simulink model "substation"  (R2023b)
settings: Solver=VariableStepAuto  StartTime=0.0  StopTime=1  FixedStep=1/48000  MaxStep=1e-3  RelTol=1e-3  EnableMultiTasking=on
libraries: spsGroundLib x4, spsThreePhaseBreakerLib x3, spsSurgeArresterLib x3, spsThreePhaseVIMeasurementLib x2, spsThreePhaseParallelRLCLoadLib x1, spsThreePhaseDynamicLoadLib x1, spsThreePhaseProgrammableVoltageSourceLib x1, dspnetwork x1, spsThreePhaseTransformerTwoWindingsLib x1, sps_lib x1
settings Model: SimulationMode=rapid-accelerator  Creator=foo  LastModifiedBy=shaow
settings SolverCC: AlgebraicLoopSolver=TrustRegion  AutoInsertRateTranBlk=on  MaxZcPerStep=1
settings DataIOCC: LimitDataPoints=on  MaxDataPoints=10000  SaveOutput=off  DSMLogging=off  SaveTime=off
settings OptimizationCC: ReuseModelBlockBuffer=off  LifeSpan=inf  SimCompilerOptimization=on
settings DebuggingCC: UnconnectedInputMsg=warning  UnconnectedOutputMsg=warning  UnconnectedLineMsg=warning  AllowSymbolicDim=off  SFUnexpectedBacktrackingDiag=warning  SFNoUnconditionalDefaultTransitionDiag=warning  SFExecutionAtInitializationDiag=none  ArithmeticOperatorsInVariantConditions=warning
settings ModelReferenceCC: EnableRefExpFcnMdlSchedulingChecks=on
settings SFSimCC: SimUseLocalCustomCode=off  CustomCodeUndefinedFunction=UseInterfaceOnly
settings RTWCC: RTWUseLocalCustomCode=off  Toolchain=MinGW64 | gmake (64-bit Windows)  BuildConfiguration=Faster Runs  DLArmComputeVersion=19.05
settings CodeAppCC: StateflowObjectComments=on
settings ConfigComp: CovMetricSettings=dw  CovSaveCumulativeToWorkspaceVar=on  CovSaveSingleToWorkspaceVar=on  CovExternalEMLEnable=off  CovSFcnEnable=off
settings SimscapeCC: SimscapeLogType=all  SimscapeLogSimulationStatistics=on  SimscapeLogDataHistory=10000

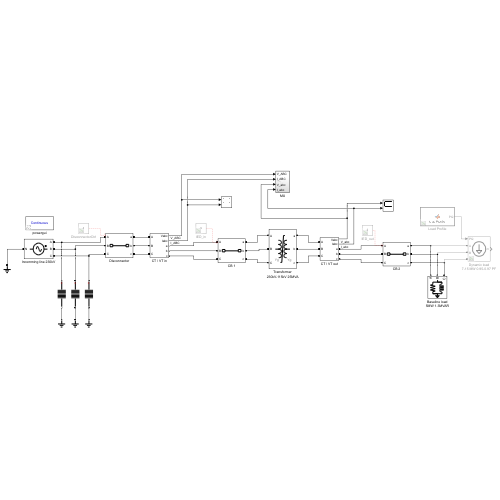
[thumbnail: Simulink's stored preview of the top-level diagram]
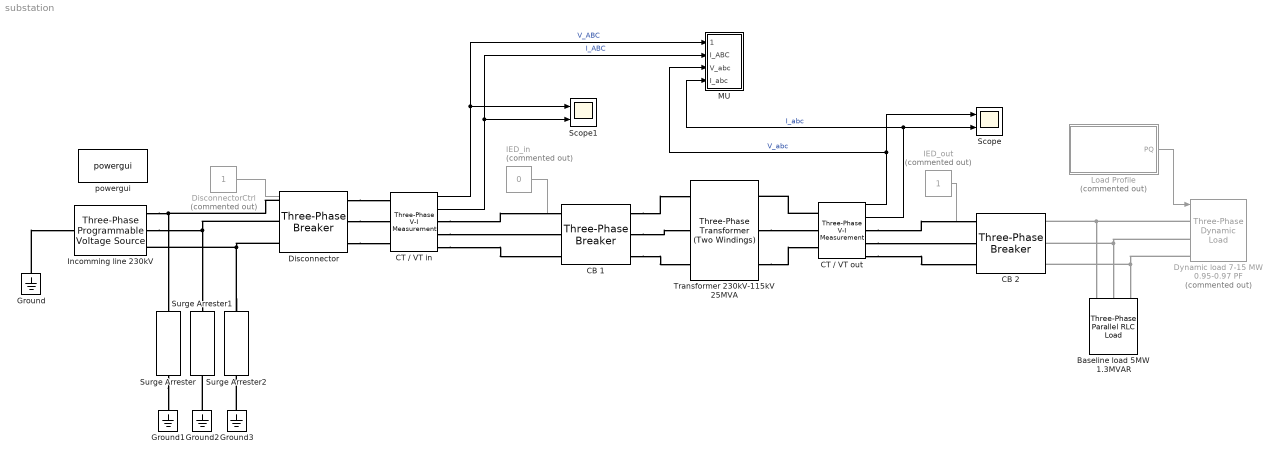
== system substation ==
  Baseline load 5MW 1.3MVAR : spsThreePhaseParallelRLCLoadLib/Three-Phase Parallel RLC Load  LConnTagsString=A|B|C  Configuration=Y (grounded)  NominalVoltage=115e3  Vabc=[1e3 1e3 1e3]  Vabcp=[1e3 1e3 1e3]  NominalFrequency=60  UnbalancedPower=off  ActivePower=24e6  InductivePower=1.3e6  CapacitivePower=0  Pabc=[10e3 9e3 11e3]  QLabc=[100 90 110]  QCabc=[100 90 110]  Pabcp=[10e3 9e3 11e3]  QLabcp=[100 90 110]  QCabcp=[100 90 110]  Measurements=None  LoadType=constant PQ
  CB 1 : spsThreePhaseBreakerLib/Three-Phase Breaker  InitialState=closed  SwitchA=on  SwitchB=on  SwitchC=on  SwitchTimes=[1e9]  External=off  BreakerResistance=0.01  SnubberResistance=1e9  SnubberCapacitance=0  Measurements=None
  CB 2 : spsThreePhaseBreakerLib/Three-Phase Breaker  InitialState=closed  SwitchA=on  SwitchB=on  SwitchC=on  SwitchTimes=[1/30]  External=off  BreakerResistance=0.01  SnubberResistance=1e9  SnubberCapacitance=0  Measurements=None
  CT / VT in : spsThreePhaseVIMeasurementLib/Three-Phase V-I Measurement  VoltageMeasurement=phase-to-phase  SetLabelV=off  LabelV=Vabc  Vpu=off  VpuLL=off  CurrentMeasurement=yes  SetLabelI=off  LabelI=Iabc  Ipu=off  Pbase=100e6  Vbase=500e3  OutputType=Complex  PhasorSimulation=off  PSBequivalent=0
  CT / VT out : spsThreePhaseVIMeasurementLib/Three-Phase V-I Measurement  VoltageMeasurement=phase-to-phase  SetLabelV=off  LabelV=Vabc  Vpu=off  VpuLL=off  CurrentMeasurement=yes  SetLabelI=off  LabelI=Iabc  Ipu=off  Pbase=100e6  Vbase=500e3  OutputType=Complex  PhasorSimulation=off  PSBequivalent=0
  Disconnector : spsThreePhaseBreakerLib/Three-Phase Breaker  InitialState=closed  SwitchA=on  SwitchB=on  SwitchC=on  SwitchTimes=[1e9]  External=off  BreakerResistance=0.01  SnubberResistance=1e9  SnubberCapacitance=0  Measurements=None
  DisconnectorCtrl : Constant  Commented=on
  Dynamic load 7-15 MW 0.95-0.97 PF : spsThreePhaseDynamicLoadLib/Three-Phase Dynamic Load  Commented=on  NominalVoltage=[115e3 60]  ActiveReactivePowers=[0 0]  PositiveSequence=[0.994 -11.8]  ExternalControl=on  NpNq=[1.3 2]  TimeConstants="[0  0  0  0]"  MinimumVoltage=0.7  Tfilter=1e-4  LoadFlowParameters=[4,0,0,0,0]
      settings: LibrarySourceBlock=|
      | sps_lib/Passives/Three-Phase
      | Dynamic Load
  Ground{,1..3} (4 alike) : spsGroundLib/Ground  LConnTagsString=a
  IED_in : Constant  Commented=on  Value=0
  IED_out : Constant  Commented=on
  Incomming line 230kV : spsThreePhaseProgrammableVoltageSourceLib/Three-Phase Programmable Voltage Source  PositiveSequence="[230e3  0 60]"  VariationEntity=None  VariationType=Step  VariationTypeAlt=Step  VariationStep=0.5  VariationRate=10  VariationMagnitude=0.3  VariationFrequency=2  VariationTiming=[1 2]  VariationPhaseA=off  Amplitudes=[1 0.8 1.2 1.0]  TimeValues=[0 0.1 0.15 0.2]  HarmonicGeneration=off  HarmonicA=[3 0.2 -25 0]  HarmonicB=[2 0.15 35 2]  Timing="[0.05  3]"  BusType=swing  Pref=50  Qref=0  Qmin=-inf  Qmax=inf
  Load Profile : MATLAB Function  Commented=on  TreatAsAtomicUnit=on  SystemSampleTime=1/2
  MU : Subsystem
  Scope : Scope  NumInputPorts=2
  Scope1 : Scope  NumInputPorts=2
  Surge Arrester : spsSurgeArresterLib/Surge Arrester  ProtectionVoltage=500e+03  Columns=2  ReferenceCurrent=500  Segment1=[.955 50]  Segment2=[1.0 25]  Segment3=[.9915 16.5]  Measurements=None  BreakLoop=off  UseDiscreteRobustSolver=on
      settings: LibrarySourceBlock=sps_lib/Passives/Surge Arrester
  Surge Arrester1 : spsSurgeArresterLib/Surge Arrester  ProtectionVoltage=500e+03  Columns=2  ReferenceCurrent=500  Segment1=[.955 50]  Segment2=[1.0 25]  Segment3=[.9915 16.5]  Measurements=None  BreakLoop=off  UseDiscreteRobustSolver=on
      settings: LibrarySourceBlock=sps_lib/Passives/Surge Arrester
  Surge Arrester2 : spsSurgeArresterLib/Surge Arrester  ProtectionVoltage=500e+03  Columns=2  ReferenceCurrent=500  Segment1=[.955 50]  Segment2=[1.0 25]  Segment3=[.9915 16.5]  Measurements=None  BreakLoop=off  UseDiscreteRobustSolver=on
      settings: LibrarySourceBlock=sps_lib/Passives/Surge Arrester
  Transformer 230kV-115kV 25MVA : spsThreePhaseTransformerTwoWindingsLib/Three-Phase Transformer (Two Windings)  Winding1Connection=Yg  Winding2Connection=Yg  CoreType=Three single-phase transformers  SetSaturation=on  Hysteresis=off  DataFile='hysteresis'  SetInitialFlux=off  Measurements=None  UNITS=pu  NominalPower=[ 25e6 , 60 ]  Winding1=[ 230e3 , 2e-3 , 8e-2 ]  Winding2=[ 115e3 , 2e-3 , 8e-2 ]  Rm=500  Lm=500  L0=0.15752  Saturation=[ 0,0 ; 0.0024,1.2 ; 1.0,1.52 ]  InitialFluxes=[-0.982867407610062 0.554941884639967 0.427925522970085]  BreakLoop=off  DiscreteSolver=Trapezoidal iterative  DataType=off  TransfoNumber=1
  powergui : sps_lib/powergui  Priority=1  SimulationMode=Continuous  SampleTime=50e-6  frequency=60  Iterations=50  frequencyindice=60  Pbase=100e6  ErrMax=1e-4  UnitsV=kV  UnitsW=MW  buscounter=0  FunctionMessages=off  echomessages=off  EnableUseOfTLC=off  CurrentSourceSwitches=off  DisableSnubberDevices=off  DisableRonSwitches=off  DisableVfSwitches=off  DisplayEquations=off  AutomaticDiscreteSolvers=on  SolverType=Tustin/Backward Euler (TBE)  Interpol=off  ExternalGateDelay=off  methode=off  Ts=100  x0status=blocks  SPID=on  SwTol=0  HookPort=off  NonlinearTolerance=1e-4  nMaxIteration=100  ContinueOnMaxIteration=off  RestoreLinks=warning  ResistiveCurrentMeasurement=off  Frange=[0:2:500]  Ylog=off  Xlog=on  ShowGrid=off  save=off  variable=ZData  structure=0  ZoomFFT=off  StartTime=0.0  cycles=1  DisplayStyle=1  fundamental=60  FreqAxis=off  MaxFrequency=1000  frequencyindicesteady=1  RmsSteady=1  display=off
  wires:
  IED_in/1 -> ?
  IED_out/1 -> ?
  DisconnectorCtrl/1 -> ?
  Load Profile/1(PQ) -> Dynamic load 7-15 MW 0.95-0.97 PF/1
  CT / VT in/1 -> Scope1/1, MU/1(V_ABC)  "V_ABC"
  CT / VT out/1 -> Scope/1, MU/3(V_abc)  "V_abc"
  CT / VT in/2 -> Scope1/2, MU/2(I_ABC)  "I_ABC"
  CT / VT out/2 -> Scope/2, MU/4(I_abc)  "I_abc"
  connections:
  Ground3/LConn1 -- Surge Arrester2/RConn1
  Ground2/LConn1 -- Surge Arrester1/RConn1
  Ground/LConn1 -- Incomming line 230kV/LConn1
  Surge Arrester/RConn1 -- Ground1/LConn1
  Surge Arrester2/LConn1 -- Disconnector/LConn3 -- Incomming line 230kV/RConn3
  Incomming line 230kV/RConn1 -- Disconnector/LConn1 -- Surge Arrester/LConn1
  Incomming line 230kV/RConn2 -- Disconnector/LConn2 -- Surge Arrester1/LConn1
  Transformer 230kV-115kV 25MVA/RConn2 -- CT / VT out/LConn2
  CT / VT out/LConn1 -- Transformer 230kV-115kV 25MVA/RConn1
  Transformer 230kV-115kV 25MVA/RConn3 -- CT / VT out/LConn3
  Disconnector/RConn1 -- CT / VT in/LConn1
  Disconnector/RConn2 -- CT / VT in/LConn2
  Disconnector/RConn3 -- CT / VT in/LConn3
  Dynamic load 7-15 MW 0.95-0.97 PF/LConn3 -- Baseline load 5MW 1.3MVAR/LConn3 -- CB 2/RConn3
  Dynamic load 7-15 MW 0.95-0.97 PF/LConn1 -- Baseline load 5MW 1.3MVAR/LConn1 -- CB 2/RConn1
  CT / VT in/RConn1 -- CB 1/LConn1
  CT / VT in/RConn2 -- CB 1/LConn2
  CT / VT in/RConn3 -- CB 1/LConn3
  CB 1/RConn1 -- Transformer 230kV-115kV 25MVA/LConn1
  CT / VT out/RConn1 -- CB 2/LConn1
  CT / VT out/RConn2 -- CB 2/LConn2
  CT / VT out/RConn3 -- CB 2/LConn3
  CB 1/RConn2 -- Transformer 230kV-115kV 25MVA/LConn2
  CB 1/RConn3 -- Transformer 230kV-115kV 25MVA/LConn3
  Dynamic load 7-15 MW 0.95-0.97 PF/LConn2 -- CB 2/RConn2 -- Baseline load 5MW 1.3MVAR/LConn2

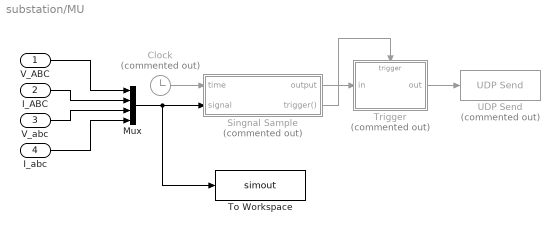
== system substation/MU ==
  V_ABC : Inport
  I_ABC : Inport  Port=2
  V_abc : Inport  Port=3
  I_abc : Inport  Port=4
  Clock : Clock  Commented=on
  Mux : Mux
  Singnal Sample : MATLAB Function  Commented=on  TreatAsAtomicUnit=on  SystemSampleTime=1/4800
  To Workspace : ToWorkspace  VariableName=simout  SaveFormat=Timeseries  SampleTime=1/4800
      settings: MaxDataPoints=4800
  Trigger : MATLAB Function  Commented=on  TreatAsAtomicUnit=on
  UDP Send : dspnetwork/UDP Send  Commented=on  remoteURL='127.0.0.1'  remotePort=9002  localURL='0.0.0.0'  localPortSource=Automatically determine  localPort=-1  sendBufferSize=65535  sampletime=-1  blockPlatform=[]  separateLengthPort=0
      settings: LibrarySourceBlock=dspsnks4/UDP Send
  wires:
  Mux/1 -> To Workspace/1, Singnal Sample/2(signal)
  Singnal Sample/2(trigger()) -> Trigger/Trigger
  Clock/1 -> Singnal Sample/1(time)
  Singnal Sample/1(output) -> Trigger/1(in)
  Trigger/1(out) -> UDP Send/1
  V_ABC/1 -> Mux/1
  I_abc/1 -> Mux/4
  I_ABC/1 -> Mux/2
  V_abc/1 -> Mux/3

== matlab function substation/Load Profile ==
  data: PQ output
function PQ = loadProfile()
    time_now = datetime('now');
    ss_of_day = time_now.Second + time_now.Minute * 60 + time_now.Hour * 3600;
    P = polyval([3.7196928531138658e-030
                -1.1470846625087270e-024
                 1.3796559275567614e-019
                -8.1199192921528985e-015
                 2.4064486502564268e-010
                -3.5099543942742386e-06
                 3.4158964141955162e-002
                -2.4634320583637030e+002
                 8.0477016798498404e+006], ss_of_day) - 10e3 * rand();
    PF = 0.97 - 1e-4 + 2e-4 * rand();
    Q = P * tan(acos(PF));
    PQ = [P, Q];

== matlab function substation/MU/Singnal Sample ==
  settings: updateMethod=DISCRETE
  data: time input; signal input; output output
  events: trigger output FUNCTION_CALL_EVENT
% This function run at 4.8 kHz, buffer 480 sample data
function output = sample(time, signal)
    % Persistent variables for the circular buffer and index
    persistent buffer sortedBuffer bufferIndex;
    if isempty(buffer)
        % Initialize the buffer
        buffer = zeros(480, 13, 'single');
        sortedBuffer = zeros(480, 13, 'single');
        bufferIndex = 1;
    end

    % Update the buffer with the new sample
    buffer(bufferIndex, :) = [...
        time,...
        signal(1), signal(2), signal(3),... % V_ABC 
        signal(4), signal(5), signal(6),... % I_ABC
        signal(7), signal(8), signal(9),... % V_abc
        signal(10), signal(11), signal(12) % I_abc
    ];
    % Increment the buffer index and wrap around if necessary
    bufferIndex = mod(bufferIndex, 480) + 1;

    % Reararnge buffer data
    if bufferIndex == 1
        % Buffer is exactly full, all data is recent
        sortedBuffer = buffer;
    else
        % Wrap around the circular buffer
        sortedBuffer(1:(480 - bufferIndex + 1), :) = buffer(bufferIndex:end, :);
        sortedBuffer((480 - bufferIndex + 2):end, :) = buffer(1:(bufferIndex - 1), :);
    end
    output = sortedBuffer;

    % Set output update flag
    persistent lastUpdateTime;
    if isempty(lastUpdateTime); lastUpdateTime = 0; end
    if time - lastUpdateTime >= 0.1
        trigger();
        lastUpdateTime = time;
    end

    % Save the last second of data to a .mat file
    %save(sprintf('signal_log/V_ABC-%.3f.mat', time), 'output');

end

== matlab function substation/MU/Trigger ==
  data: in input; out output
  events: trigger input FUNCTION_CALL_EVENT
function out = passthrough(in)
%#codegen

out = in;
